simulink model "SeatMdSwtchArbt"  (R2018b)
settings: Solver=FixedStepDiscrete  StartTime=0.0  StopTime=10.0  FixedStep=0.01  RelTol=1e-3
undefined symbols (not defined in the file or in its folder): PosRclRspStat1
libraries: SeatMdSwtchArbt_Lib x35
(part 2 of 2)

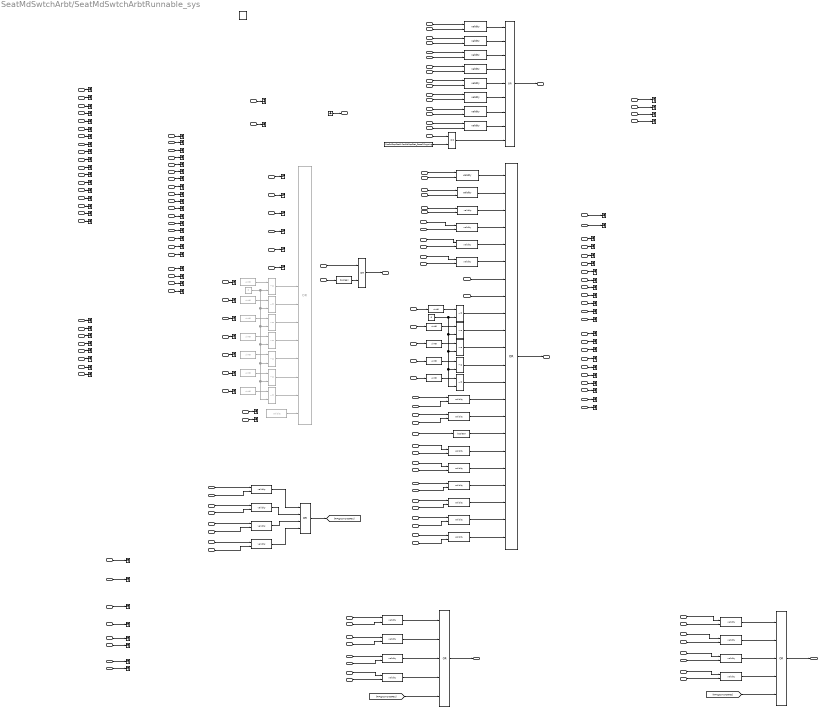
== system SeatMdSwtchArbt/SeatMdSwtchArbtRunnable_sys ==
  note: 2022-02-17:CR202175：修改需求506/548/551/552，新增需求712，完善座椅模式的打断策略。
      | 2023-07-31:增加2L/2R腿托无极调节接口
  note: #尾箱靠背调节
  note: #尾箱前后调节
  note: #坐垫折叠
  IfDrvSeatMemSwtAct1_Val_read : Inport
  IfDrvSeatMemSwtActV1_Val_read : Inport  Port=2
  IfVeSMSb_DrvStCshnRrDnwdMovSwAct_Val_read : Inport  Port=3
  IfVeSMSb_DrvStCshnRrDnwdMovSwActV_Val_read : Inport  Port=4
  IfVeSMSb2LBkReclnSwReq_Val_read : Inport  Port=5
  IfVeSMSb2LBkReclnSwReqV_Val_read : Inport  Port=6
  IfVeSMSb2LSecRwStBkReclnDnwdSwActv_Val_read : Inport  Port=7
  IfVeSMSb2LSecRwStBkReclnUpwdSwActv_Val_read : Inport  Port=8
  IfVeSMSb2LSecRwStBkwdSwActv_Val_read : Inport  Port=9
  IfVeSMSb2LSecRwStFrwdSwActv_Val_read : Inport  Port=10
  IfVeSMSb2LSecRwStLgrstDnwdSwActv_Val_read : Inport  Port=11
  IfVeSMSb2LSecRwStLgrstUpwdSwActv_Val_read : Inport  Port=12
  IfVeSMSbBosSWBkwdHMI2RReq_Val_read : Inport  Port=13
  IfVeSMSbBosSWFrwdHMI2RReq_Val_read : Inport  Port=14
  IfVeSMSbBosSWStBkReclnDnwdHMI2RReq_Val_read : Inport  Port=15
  IfVeSMSbBosSWStBkReclnUpwdHMI2RReq_Val_read : Inport  Port=16
  IfVeSMSbDrvStBkReclnDnwdMovSwAct_Val_read : Inport  Port=17
  IfVeSMSbDrvStBkReclnDnwdMovSwActV_Val_read : Inport  Port=18
  IfVeSMSbDrvStBkReclnUpwdMovSwAct_Val_read : Inport  Port=19
  IfVeSMSbDrvStBkReclnUpwdMovSwActV_Val_read : Inport  Port=20
  IfVeSMSbDrvStBkwdMovSwAct_Val_read : Inport  Port=21
  IfVeSMSbDrvStBkwdMovSwActV_Val_read : Inport  Port=22
  IfVeSMSbDrvStCshnFrntDnwdMovSwAct_Val_read : Inport  Port=23
  IfVeSMSbDrvStCshnFrntDnwdMovSwActV_Val_read : Inport  Port=24
  IfVeSMSbDrvStCshnFrntUpwdMovSwAct_Val_read : Inport  Port=25
  IfVeSMSbDrvStCshnFrntUpwdMovSwActV_Val_read : Inport  Port=26
  IfVeSMSbDrvStCshnRrUpwdMovSwAct_Val_read : Inport  Port=27
  IfVeSMSbDrvStCshnRrUpwdMovSwActV_Val_read : Inport  Port=28
  IfVeSMSbDrvStFrwdMovSwAct_Val_read : Inport  Port=29
  IfVeSMSbDrvStFrwdMovSwActV_Val_read : Inport  Port=30
  IfVeSMSbPassStBkReclnDnwdMovSwAct_Val_read : Inport  Port=31
  IfVeSMSbPassStBkReclnDnwdMovSwActV_Val_read : Inport  Port=32
  IfVeSMSbPassStBkReclnUpwdMovSwAct_Val_read : Inport  Port=33
  IfVeSMSbPassStBkReclnUpwdMovSwActV_Val_read : Inport  Port=34
  IfVeSMSbPassStBkwdMovSwAct_Val_read : Inport  Port=35
  IfVeSMSbPassStBkwdMovSwActV_Val_read : Inport  Port=36
  IfVeSMSbPassStCshnFrntDnwdMovSwAct_Val_read : Inport  Port=37
  IfVeSMSbPassStCshnFrntDnwdMovSwActV_Val_read : Inport  Port=38
  IfVeSMSbPassStCshnFrntUpwdMovSwAct_Val_read : Inport  Port=39
  IfVeSMSbPassStCshnFrntUpwdMovSwActV_Val_read : Inport  Port=40
  IfVeSMSbPassStCshnRrDnwdMovSwAct_Val_read : Inport  Port=41
  IfVeSMSbPassStCshnRrDnwdMovSwActV_Val_read : Inport  Port=42
  IfVeSMSbPassStCshnRrUpwdMovSwAct_Val_read : Inport  Port=43
  IfVeSMSbPassStCshnRrUpwdMovSwActV_Val_read : Inport  Port=44
  IfVeSMSbPassStFrwdMovSwAct_Val_read : Inport  Port=45
  IfVeSMSbPassStFrwdMovSwActV_Val_read : Inport  Port=46
  IfVeSMSbRrLtStFtDnwdHMI2LReq_Val_read : Inport  Port=47
  IfVeSMSbRrLtStFtUpwdHMI2LReq_Val_read : Inport  Port=48
  IfVeSMSbRrPsgComprtStBkReclnDnwdSwReq_Val_read : Inport  Port=49
  IfVeSMSbRrPsgComprtStBkReclnDnwdSwReqV_Val_read : Inport  Port=50
  IfVeSMSbRrPsgComprtStBkReclnUpwdSwReq_Val_read : Inport  Port=51
  IfVeSMSbRrPsgComprtStBkReclnUpwdSwReqV_Val_read : Inport  Port=52
  IfVeSMSbRrPsgComprtStBkwdSwReq_Val_read : Inport  Port=53
  IfVeSMSbRrPsgComprtStBkwdSwReqV_Val_read : Inport  Port=54
  IfVeSMSbRrPsgComprtStFrwdSwReq_Val_read : Inport  Port=55
  IfVeSMSbRrPsgComprtStFrwdSwReqV_Val_read : Inport  Port=56
  IfVeSMSbRrRtStFtDnwdHMI2RReq_Val_read : Inport  Port=57
  IfVeSMSbRrRtStFtUpwdHMI2RReq_Val_read : Inport  Port=58
  IfVeSMSbSecRwLtStArmScrnHMI2LReq_Val_read : Inport  Port=59
  IfVeSMSbSecRwLtStBkReclnDnwdHMI2LReq_Val_read : Inport  Port=60
  IfVeSMSbSecRwLtStBkReclnUpwdHMI2LReq_Val_read : Inport  Port=61
  IfVeSMSbSecRwLtStBkwdHMI2LReq_Val_read : Inport  Port=62
  IfVeSMSbSecRwLtStFrwdHMI2LReq_Val_read : Inport  Port=63
  IfVeSMSbSecRwLtStFtDnwdHMI2LReq_Val_read : Inport  Port=64
  IfVeSMSbSecRwLtStFtUpwdHMI2LReq_Val_read : Inport  Port=65
  IfVeSMSbSecRwLtStHdrstBkwdHMI2LReq_Val_read : Inport  Port=66
  IfVeSMSbSecRwLtStHdrstDnwdHMI2LReq_Val_read : Inport  Port=67
  IfVeSMSbSecRwLtStHdrstFrwdHMI2LReq_Val_read : Inport  Port=68
  IfVeSMSbSecRwLtStHdrstUpwdHMI2LReq_Val_read : Inport  Port=69
  IfVeSMSbSecRwLtStLcMovActv_Val_read : Inport  Port=70
  IfVeSMSbSecRwLtStLgrstDnwdHMI2LReq_Val_read : Inport  Port=71
  IfVeSMSbSecRwLtStLgrstInwdHMI2LReq_Val_read : Inport  Port=72
  IfVeSMSbSecRwLtStLgrstOtwdHMI2LReq_Val_read : Inport  Port=73
  IfVeSMSbSecRwLtStLgrstUpwdHMI2LReq_Val_read : Inport  Port=74
  IfVeSMSbSecRwLtStLtwdHMI2LReq_Val_read : Inport  Port=75
  IfVeSMSbSecRwLtStRtwdHMI2LReq_Val_read : Inport  Port=76
  IfVeSMSbSecRwRtStArmScrnHMI2RReq_Val_read : Inport  Port=77
  IfVeSMSbSecRwRtStBkReclnDnwdHMI2RReq_Val_read : Inport  Port=78
  IfVeSMSbSecRwRtStBkReclnDnwdSwReq_Val_read : Inport  Port=79
  IfVeSMSbSecRwRtStBkReclnDnwdSwReqV_Val_read : Inport  Port=80
  IfVeSMSbSecRwRtStBkReclnUpwdHMI2RReq_Val_read : Inport  Port=81
  IfVeSMSbSecRwRtStBkReclnUpwdSwReq_Val_read : Inport  Port=82
  IfVeSMSbSecRwRtStBkReclnUpwdSwReqV_Val_read : Inport  Port=83
  IfVeSMSbSecRwRtStBkwdHMI2RReq_Val_read : Inport  Port=84
  IfVeSMSbSecRwRtStBkwdSwReq_Val_read : Inport  Port=85
  IfVeSMSbSecRwRtStBkwdSwReqV_Val_read : Inport  Port=86
  IfVeSMSbSecRwRtStFrwdHMI2RReq_Val_read : Inport  Port=87
  IfVeSMSbSecRwRtStFrwdSwReq_Val_read : Inport  Port=88
  IfVeSMSbSecRwRtStFrwdSwReqV_Val_read : Inport  Port=89
  IfVeSMSbSecRwRtStFtDnwdHMI2RReq_Val_read : Inport  Port=90
  IfVeSMSbSecRwRtStFtUpwdHMI2RReq_Val_read : Inport  Port=91
  IfVeSMSbSecRwRtStHdrstBkwdHMI2RReq_Val_read : Inport  Port=92
  IfVeSMSbSecRwRtStHdrstDnwdHMI2RReq_Val_read : Inport  Port=93
  IfVeSMSbSecRwRtStHdrstFrwdHMI2RReq_Val_read : Inport  Port=94
  IfVeSMSbSecRwRtStHdrstUpwdHMI2RReq_Val_read : Inport  Port=95
  IfVeSMSbSecRwRtStLgrstDnwdHMI2RReq_Val_read : Inport  Port=96
  IfVeSMSbSecRwRtStLgrstDnwdSwReq_Val_read : Inport  Port=97
  IfVeSMSbSecRwRtStLgrstDnwdSwReqV_Val_read : Inport  Port=98
  IfVeSMSbSecRwRtStLgrstInwdHMI2RReq_Val_read : Inport  Port=99
  IfVeSMSbSecRwRtStLgrstOtwdHMI2RReq_Val_read : Inport  Port=100
  IfVeSMSbSecRwRtStLgrstUpwdHMI2RReq_Val_read : Inport  Port=101
  IfVeSMSbSecRwRtStLgrstUpwdSwReq_Val_read : Inport  Port=102
  IfVeSMSbSecRwRtStLgrstUpwdSwReqV_Val_read : Inport  Port=103
  IfVeSMSbSecRwRtStLmbrHMI2RReq_Val_read : Inport  Port=104
  IfVeSMSbSecRwRtStLtwdHMI2RReq_Val_read : Inport  Port=105
  IfVeSMSbSecRwRtStRtwdHMI2RReq_Val_read : Inport  Port=106
  IfVeSMSbThdRLtStExpdSwReq_Val_read : Inport  Port=107
  IfVeSMSbThdRLtStExpdSwReqV_Val_read : Inport  Port=108
  IfVeSMSbThdRRtStExpdSwReq_Val_read : Inport  Port=109
  IfVeSMSbThdRRtStExpdSwReqV_Val_read : Inport  Port=110
  IfVeSMSbThdRwLtStBkReclnDnwdSwReq_Val_read : Inport  Port=111
  IfVeSMSbThdRwLtStBkReclnDnwdSwReqV_Val_read : Inport  Port=112
  IfVeSMSbThdRwLtStBkReclnUpwdSwReq_Val_read : Inport  Port=113
  IfVeSMSbThdRwLtStBkReclnUpwdSwReqV_Val_read : Inport  Port=114
  IfVeSMSbThdRwLtStBkwdSwReq_Val_read : Inport  Port=115
  IfVeSMSbThdRwLtStBkwdSwReqV_Val_read : Inport  Port=116
  IfVeSMSbThdRwLtStFrwdSwReq_Val_read : Inport  Port=117
  IfVeSMSbThdRwLtStFrwdSwReqV_Val_read : Inport  Port=118
  IfVeSMSbThdRwRtStBkReclnDnwdSwReq_Val_read : Inport  Port=119
  IfVeSMSbThdRwRtStBkReclnDnwdSwReqV_Val_read : Inport  Port=120
  IfVeSMSbThdRwRtStBkReclnUpwdSwReq_Val_read : Inport  Port=121
  IfVeSMSbThdRwRtStBkReclnUpwdSwReqV_Val_read : Inport  Port=122
  IfVeSMSbThdRwRtStBkwdSwReq_Val_read : Inport  Port=123
  IfVeSMSbThdRwRtStBkwdSwReqV_Val_read : Inport  Port=124
  IfVeSMSbThdRwRtStFrwdSwReq_Val_read : Inport  Port=125
  IfVeSMSbThdRwRtStFrwdSwReqV_Val_read : Inport  Port=126
  IfVeSMSeSecLTMemHMI2LReq1_Val_read : Inport  Port=127
  IfVeSMSeSecLTMemHMI2RReq1_Val_read : Inport  Port=128
  IfVeSMSuSeatPosEnable_Val_read : Inport  Port=129
  StSlctSwReq_Val_read : Inport  Port=130
  StSlctSwReqV_Val_read : Inport  Port=131
  IfVeSMSuRrLtStFtUpwdPstnHMI2LReq_Val_read : Inport  Port=132
  IfVeSMSuRrLtStFtUpwdPstnHMI2LReqV_Val_read : Inport  Port=133
  IfVeSMSuRrRtStFtUpwdPstnHMI2RReq_Val_read : Inport  Port=134
  IfVeSMSuRrRtStFtUpwdPstnHMI2RReqV_Val_read : Inport  Port=135
  IfVeSMSbSecRwLtStFtClsHMI2LReq_Val_read : Inport  Port=136
  IfVeSMSbSecRwLtStFtOpenHMI2LReq_Val_read : Inport  Port=137
  IfVeSMSbSecRwRtStFtClsHMI2LReq_Val_read : Inport  Port=138
  IfVeSMSbSecRwRtStFtOpenHMI2LReq_Val_read : Inport  Port=139
  IfSecRwLtStCushnFrtDnwdHMI2LReq_Val_read : Inport  Port=140
  IfSecRwLtStCushnFrtUpwdDnwdMovmtVirtCtrlReq_Val_read : Inport  Port=141
  IfSecRwLtStCushnFrtUpwdHMI2LReq_Val_read : Inport  Port=142
  IfSecRwLtStFwdBkwdMovmtVirtCtrlReq_Val_read : Inport  Port=143
  IfSecRwLtStLgrstOtwdInwdMovmtVirtCtrlReq_Val_read : Inport  Port=144
  IfSecRwLtStLgrstUpwdDnwdMovmtVirtCtrlReq_Val_read : Inport  Port=145
  IfSecRwLtStRclUpwdDnwdMovmtVirtCtrlReq_Val_read : Inport  Port=146
  IfSecRwRtStCushnFrtDnwdHMI2LReq_Val_read : Inport  Port=147
  IfSecRwRtStCushnFrtUpwdDnwdMovmtVirtCtrlReq_Val_read : Inport  Port=148
  IfSecRwRtStCushnFrtUpwdHMI2LReq_Val_read : Inport  Port=149
  IfSecRwRtStFwdBkwdMovmtVirtCtrlReq_Val_read : Inport  Port=150
  IfSecRwRtStLgrstOtwdInwdMovmtVirtCtrlReq_Val_read : Inport  Port=151
  IfSecRwRtStLgrstUpwdDnwdMovmtVirtCtrlReq_Val_read : Inport  Port=152
  IfSecRwRtStRclUpwdDnwdMovmtVirtCtrlReq_Val_read : Inport  Port=153
  IfSecRwRtStLgrstInwdSwReq_Val_read : Inport  Port=154
  IfSecRwRtStLgrstInwdSwReqV_Val_read : Inport  Port=155
  IfSecRwRtStLgrstOtwdSwReq_Val_read : Inport  Port=156
  IfSecRwRtStLgrstOtwdSwReqV_Val_read : Inport  Port=157
  IfVeSMSbPassStBkReclnDnwdMovBosSwAct_Val_read : Inport  Port=158
  IfVeSMSbPassStBkReclnDnwdMovBosSwActV_Val_read : Inport  Port=159
  IfVeSMSbPassStBkReclnUpwdMovBosSwAct_Val_read : Inport  Port=160
  IfVeSMSbPassStBkReclnUpwdMovBosSwActV_Val_read : Inport  Port=161
  IfVeSMSbPassStBkwdMovBosSwAct_Val_read : Inport  Port=162
  IfVeSMSbPassStBkwdMovBosSwActV_Val_read : Inport  Port=163
  IfVeSMSbPassStFrwdMovBosSwAct_Val_read : Inport  Port=164
  IfVeSMSbPassStFrwdMovBosSwActV_Val_read : Inport  Port=165
  IfSecRwRtStZeroGrvyDnwdSwReq_Val_read : Inport  Port=166
  IfSecRwRtStZeroGrvyDnwdSwReqV_Val_read : Inport  Port=167
  IfSecRwRtStZeroGrvyUpwdSwReq_Val_read : Inport  Port=168
  IfSecRwRtStZeroGrvyUpwdSwReqV_Val_read : Inport  Port=169
  SecRwRtStBkReclnDnwdMovBossSwReq_Val_read : Inport  Port=170
  SecRwRtStBkReclnDnwdMovBossSwReqV_Val_read : Inport  Port=171
  SecRwRtStBkReclnUpwdMovBossSwReq_Val_read : Inport  Port=172
  SecRwRtStBkReclnUpwdMovBossSwReqV_Val_read : Inport  Port=173
  SecRwRtStBkwdMovBossSwReq_Val_read : Inport  Port=174
  SecRwRtStBkwdMovBossSwReqV_Val_read : Inport  Port=175
  SecRwRtStFrwdMovBossSwReq_Val_read : Inport  Port=176
  SecRwRtStFrwdMovBossSwReqV_Val_read : Inport  Port=177
  PassStPosRclRspStat_Val_read : Inport  Port=178
  function : TriggerPort  TriggerType=function-call  VariantControl=(inherit)  SampleTimeType=periodic  SampleTime=-1
  AND : Logic  Operator=OR  Inputs=9  AllPortsSameDT=off  OutDataTypeStr=boolean
  Constant1 : Constant  Value=PosRclRspStat1.PosRclRspStat_RecallOngoing  OutDataTypeStr=Enum:PosRclRspStat1
  Constant2 : Constant  Commented=on  Value=0  OutDataTypeStr=uint8
  Constant3 : Constant  Value=0  OutDataTypeStr=uint8
  Data Type Conversion{,1..6} (7 alike) : DataTypeConversion  Commented=on  OutDataTypeStr=uint8
  Data Type Conversion{7..9,11,13} (5 alike) : DataTypeConversion  OutDataTypeStr=uint8
  Data Type Conversion14 : DataTypeConversion  OutDataTypeStr=boolean
  Data Type Conversion15 : DataTypeConversion  OutDataTypeStr=boolean
  Equal{,1..6} (7 alike) : RelationalOperator  Commented=on  Operator=~=  OutDataTypeStr=boolean  RndMeth=Simplest
  Equal10 : RelationalOperator  Operator===  OutDataTypeStr=boolean  RndMeth=Simplest
  Equal{7..9,11,13} (5 alike) : RelationalOperator  Operator=~=  OutDataTypeStr=boolean  RndMeth=Simplest
  Ground : Ground
  Logical Operator1 : Logic  Operator=OR  Inputs=5  AllPortsSameDT=off  OutDataTypeStr=boolean
  Logical Operator19 : Logic  Commented=on  Operator=OR  Inputs=14  AllPortsSameDT=off  OutDataTypeStr=boolean
  Logical Operator26 : Logic  Operator=OR  Inputs=22  AllPortsSameDT=off  OutDataTypeStr=boolean
  Logical Operator27 : Logic  Operator=OR  Inputs=5  AllPortsSameDT=off  OutDataTypeStr=boolean
  OR : Logic  Operator=OR  AllPortsSameDT=off  OutDataTypeStr=boolean
  OR1 : Logic  Operator=OR  Inputs=4  AllPortsSameDT=off  OutDataTypeStr=boolean
  Terminator_{1..34,37..44,47..69,71..72,74..82,84..105,129} (99 alike) : Terminator
  validity{1..6,8..35} (34 alike) : SeatMdSwtchArbt_Lib/validity  SystemSampleTime=-1
  validity7 : SeatMdSwtchArbt_Lib/validity  Commented=on  SystemSampleTime=-1
  IfVeSMSbIs2LStSwAct_Val_write : Outport
  IfVeSMSbIs2RStSwAct_Val_write : Outport  Port=2
  IfVeSMSbIs3LStSwAct_Val_write : Outport  Port=3
  IfVeSMSbIs3RStSwAct_Val_write : Outport  Port=4
  IfVeSMSbIsDrvStSwAct_Val_write : Outport  Port=5
  IfVeSMSbIsPasStSwAct_Val_write : Outport  Port=6
  wires:
  IfDrvSeatMemSwtAct1_Val_read/1 -> Terminator_1/1
  IfDrvSeatMemSwtActV1_Val_read/1 -> Terminator_2/1
  IfVeSMSb_DrvStCshnRrDnwdMovSwAct_Val_read/1 -> Terminator_3/1
  IfVeSMSb_DrvStCshnRrDnwdMovSwActV_Val_read/1 -> Terminator_4/1
  IfVeSMSbDrvStBkReclnDnwdMovSwAct_Val_read/1 -> Terminator_17/1
  IfVeSMSbDrvStBkReclnDnwdMovSwActV_Val_read/1 -> Terminator_18/1
  IfVeSMSbDrvStBkReclnUpwdMovSwAct_Val_read/1 -> Terminator_19/1
  IfVeSMSbDrvStBkReclnUpwdMovSwActV_Val_read/1 -> Terminator_20/1
  IfVeSMSbDrvStBkwdMovSwAct_Val_read/1 -> Terminator_21/1
  IfVeSMSbDrvStBkwdMovSwActV_Val_read/1 -> Terminator_22/1
  IfVeSMSbDrvStCshnFrntDnwdMovSwAct_Val_read/1 -> Terminator_23/1
  IfVeSMSbDrvStCshnFrntDnwdMovSwActV_Val_read/1 -> Terminator_24/1
  IfVeSMSbDrvStCshnFrntUpwdMovSwAct_Val_read/1 -> Terminator_25/1
  IfVeSMSbDrvStCshnFrntUpwdMovSwActV_Val_read/1 -> Terminator_26/1
  IfVeSMSbDrvStCshnRrUpwdMovSwAct_Val_read/1 -> Terminator_27/1
  IfVeSMSbDrvStCshnRrUpwdMovSwActV_Val_read/1 -> Terminator_28/1
  IfVeSMSbDrvStFrwdMovSwAct_Val_read/1 -> Terminator_29/1
  IfVeSMSbDrvStFrwdMovSwActV_Val_read/1 -> Terminator_30/1
  IfVeSMSbPassStCshnFrntDnwdMovSwAct_Val_read/1 -> Terminator_37/1
  IfVeSMSbPassStCshnFrntDnwdMovSwActV_Val_read/1 -> Terminator_38/1
  IfVeSMSbPassStCshnFrntUpwdMovSwAct_Val_read/1 -> Terminator_39/1
  IfVeSMSbPassStCshnFrntUpwdMovSwActV_Val_read/1 -> Terminator_40/1
  IfVeSMSbPassStCshnRrDnwdMovSwAct_Val_read/1 -> Terminator_41/1
  IfVeSMSbPassStCshnRrDnwdMovSwActV_Val_read/1 -> Terminator_42/1
  IfVeSMSbPassStCshnRrUpwdMovSwAct_Val_read/1 -> Terminator_43/1
  IfVeSMSbPassStCshnRrUpwdMovSwActV_Val_read/1 -> Terminator_44/1
  IfVeSMSbSecRwRtStLmbrHMI2RReq_Val_read/1 -> Terminator_104/1
  IfVeSMSuSeatPosEnable_Val_read/1 -> Terminator_129/1
  Ground/1 -> IfVeSMSbIsDrvStSwAct_Val_write/1
  IfVeSMSbSecRwRtStBkReclnUpwdSwReqV_Val_read/1 -> validity19/2
  IfVeSMSbSecRwRtStLgrstDnwdSwReqV_Val_read/1 -> validity22/2
  IfVeSMSbSecRwRtStFrwdSwReq_Val_read/1 -> validity21/1
  IfVeSMSbSecRwRtStLgrstUpwdSwReq_Val_read/1 -> validity23/1
  IfVeSMSbSecRwRtStBkReclnUpwdSwReq_Val_read/1 -> validity19/1
  IfVeSMSbSecRwRtStLgrstUpwdSwReqV_Val_read/1 -> validity23/2
  IfVeSMSbSecRwRtStFrwdSwReqV_Val_read/1 -> validity21/2
  Logical Operator26/1 -> IfVeSMSbIs2RStSwAct_Val_write/1
  IfVeSMSbSecRwRtStBkReclnDnwdSwReq_Val_read/1 -> validity18/1
  IfVeSMSbSecRwRtStBkReclnDnwdSwReqV_Val_read/1 -> validity18/2
  IfVeSMSbSecRwRtStBkwdSwReq_Val_read/1 -> validity20/1
  IfVeSMSbSecRwRtStBkwdSwReqV_Val_read/1 -> validity20/2
  IfVeSMSbSecRwRtStLgrstDnwdSwReq_Val_read/1 -> validity22/1
  IfVeSMSbRrPsgComprtStBkReclnDnwdSwReq_Val_read/1 -> validity3/1
  validity5/1 -> OR1/3
  IfVeSMSbRrPsgComprtStBkReclnDnwdSwReqV_Val_read/1 -> validity3/2
  validity4/1 -> OR1/2
  IfVeSMSbRrPsgComprtStFrwdSwReqV_Val_read/1 -> validity6/2
  IfVeSMSbRrPsgComprtStBkwdSwReqV_Val_read/1 -> validity5/2
  IfVeSMSbRrPsgComprtStFrwdSwReq_Val_read/1 -> validity6/1
  IfVeSMSbRrPsgComprtStBkReclnUpwdSwReq_Val_read/1 -> validity4/1
  IfVeSMSbRrPsgComprtStBkwdSwReq_Val_read/1 -> validity5/1
  validity6/1 -> OR1/4
  OR1/1 -> [RrPsgComprtStReq]
  validity3/1 -> OR1/1
  IfVeSMSbRrPsgComprtStBkReclnUpwdSwReqV_Val_read/1 -> validity4/2
  validity27/1 -> Logical Operator27/4
  IfVeSMSbThdRwLtStBkReclnUpwdSwReq_Val_read/1 -> validity25/1
  IfVeSMSbThdRwLtStBkReclnDnwdSwReqV_Val_read/1 -> validity24/2
  validity24/1 -> Logical Operator27/1
  IfVeSMSbThdRwLtStBkReclnDnwdSwReq_Val_read/1 -> validity24/1
  IfVeSMSbThdRwLtStFrwdSwReqV_Val_read/1 -> validity27/2
  IfVeSMSbThdRwLtStBkReclnUpwdSwReqV_Val_read/1 -> validity25/2
  IfVeSMSbThdRwLtStFrwdSwReq_Val_read/1 -> validity27/1
  validity25/1 -> Logical Operator27/2
  IfVeSMSbThdRwLtStBkwdSwReq_Val_read/1 -> validity26/1
  validity26/1 -> Logical Operator27/3
  Logical Operator27/1 -> IfVeSMSbIs3LStSwAct_Val_write/1
  IfVeSMSbThdRwLtStBkwdSwReqV_Val_read/1 -> validity26/2
  validity17/1 -> Logical Operator1/1
  IfVeSMSbThdRwRtStBkReclnDnwdSwReqV_Val_read/1 -> validity17/2
  validity30/1 -> Logical Operator1/4
  validity29/1 -> Logical Operator1/3
  IfVeSMSbThdRwRtStBkReclnUpwdSwReq_Val_read/1 -> validity28/1
  IfVeSMSbThdRwRtStBkwdSwReq_Val_read/1 -> validity29/1
  IfVeSMSbThdRwRtStBkReclnDnwdSwReq_Val_read/1 -> validity17/1
  IfVeSMSbThdRwRtStBkReclnUpwdSwReqV_Val_read/1 -> validity28/2
  validity28/1 -> Logical Operator1/2
  IfVeSMSbThdRwRtStFrwdSwReq_Val_read/1 -> validity30/1
  Logical Operator1/1 -> IfVeSMSbIs3RStSwAct_Val_write/1
  IfVeSMSbThdRwRtStBkwdSwReqV_Val_read/1 -> validity29/2
  IfVeSMSbThdRwRtStFrwdSwReqV_Val_read/1 -> validity30/2
  StSlctSwReq_Val_read/1 -> Terminator_5/1
  StSlctSwReqV_Val_read/1 -> Terminator_6/1
  IfVeSMSbSecRwLtStFtDnwdHMI2LReq_Val_read/1 -> Terminator_11/1
  IfVeSMSbSecRwLtStFtUpwdHMI2LReq_Val_read/1 -> Terminator_12/1
  IfVeSMSbSecRwRtStFtDnwdHMI2RReq_Val_read/1 -> Terminator_13/1
  IfVeSMSbSecRwRtStFtUpwdHMI2RReq_Val_read/1 -> Terminator_14/1
  IfVeSMSbSecRwLtStBkReclnDnwdHMI2LReq_Val_read/1 -> Terminator_15/1
  IfVeSMSbSecRwLtStBkReclnUpwdHMI2LReq_Val_read/1 -> Terminator_16/1
  IfVeSMSbSecRwLtStFrwdHMI2LReq_Val_read/1 -> Terminator_54/1
  IfVeSMSbSecRwLtStBkwdHMI2LReq_Val_read/1 -> Terminator_47/1
  IfVeSMSbSecRwLtStHdrstUpwdHMI2LReq_Val_read/1 -> Terminator_51/1
  IfVeSMSbSecRwLtStHdrstDnwdHMI2LReq_Val_read/1 -> Terminator_62/1
  IfVeSMSbSecRwLtStLgrstUpwdHMI2LReq_Val_read/1 -> Terminator_63/1
  IfVeSMSbSecRwLtStLgrstDnwdHMI2LReq_Val_read/1 -> Terminator_64/1
  IfVeSMSbSecRwLtStLtwdHMI2LReq_Val_read/1 -> Terminator_53/1
  IfVeSMSbSecRwLtStRtwdHMI2LReq_Val_read/1 -> Terminator_65/1
  IfVeSMSbRrLtStFtDnwdHMI2LReq_Val_read/1 -> Terminator_66/1
  IfVeSMSbRrLtStFtUpwdHMI2LReq_Val_read/1 -> Terminator_67/1
  IfVeSMSbSecRwLtStHdrstBkwdHMI2LReq_Val_read/1 -> Terminator_68/1
  IfVeSMSbSecRwLtStHdrstFrwdHMI2LReq_Val_read/1 -> Terminator_69/1
  IfVeSMSbSecRwLtStLgrstInwdHMI2LReq_Val_read/1 -> Terminator_71/1
  IfVeSMSbSecRwLtStLgrstOtwdHMI2LReq_Val_read/1 -> Terminator_72/1
  IfVeSMSbSecRwLtStArmScrnHMI2LReq_Val_read/1 -> Terminator_52/1
  IfVeSMSuRrLtStFtUpwdPstnHMI2LReq_Val_read/1 -> Terminator_74/1
  IfVeSMSuRrLtStFtUpwdPstnHMI2LReqV_Val_read/1 -> Terminator_75/1
  IfVeSMSbSecRwLtStFtOpenHMI2LReq_Val_read/1 -> Terminator_76/1
  IfVeSMSbSecRwLtStFtClsHMI2LReq_Val_read/1 -> Terminator_77/1
  Equal/1 -> Logical Operator19/7
  Constant2/1 -> Equal2/2, Equal6/2, Equal5/2, Equal4/2, Equal3/2, Equal1/2, Equal/2
  Equal1/1 -> Logical Operator19/8
  Equal2/1 -> Logical Operator19/9
  Equal3/1 -> Logical Operator19/10
  validity7/1 -> Logical Operator19/14
  Equal6/1 -> Logical Operator19/13
  Equal5/1 -> Logical Operator19/12
  Equal4/1 -> Logical Operator19/11
  IfVeSMSbSecRwRtStArmScrnHMI2RReq_Val_read/1 -> Terminator_48/1
  IfVeSMSbSecRwRtStBkReclnUpwdHMI2RReq_Val_read/1 -> Terminator_49/1
  IfVeSMSbSecRwRtStBkReclnDnwdHMI2RReq_Val_read/1 -> Terminator_50/1
  IfVeSMSbSecRwRtStBkwdHMI2RReq_Val_read/1 -> Terminator_61/1
  IfVeSMSbSecRwRtStFrwdHMI2RReq_Val_read/1 -> Terminator_78/1
  validity18/1 -> Logical Operator26/1
  validity19/1 -> Logical Operator26/2
  validity20/1 -> Logical Operator26/3
  validity21/1 -> Logical Operator26/4
  validity22/1 -> Logical Operator26/5
  validity23/1 -> Logical Operator26/6
  Constant3/1 -> Equal13/2, Equal11/2, Equal9/2, Equal8/2, Equal7/2
  IfVeSMSbSecRwRtStHdrstDnwdHMI2RReq_Val_read/1 -> Terminator_58/1
  IfVeSMSbSecRwRtStHdrstUpwdHMI2RReq_Val_read/1 -> Terminator_79/1
  IfVeSMSbSecRwRtStLgrstDnwdHMI2RReq_Val_read/1 -> Terminator_80/1
  IfVeSMSbSecRwRtStLgrstUpwdHMI2RReq_Val_read/1 -> Terminator_81/1
  IfVeSMSbSecRwRtStLtwdHMI2RReq_Val_read/1 -> Terminator_60/1
  IfVeSMSbSecRwRtStRtwdHMI2RReq_Val_read/1 -> Terminator_82/1
  IfVeSMSbRrRtStFtDnwdHMI2RReq_Val_read/1 -> Terminator_84/1
  IfVeSMSbRrRtStFtUpwdHMI2RReq_Val_read/1 -> Terminator_85/1
  IfVeSMSbSecRwRtStHdrstBkwdHMI2RReq_Val_read/1 -> Terminator_86/1
  IfVeSMSbSecRwRtStHdrstFrwdHMI2RReq_Val_read/1 -> Terminator_87/1
  IfVeSMSbSecRwRtStLgrstInwdHMI2RReq_Val_read/1 -> Terminator_88/1
  IfVeSMSbSecRwRtStLgrstOtwdHMI2RReq_Val_read/1 -> Terminator_89/1
  IfVeSMSuRrRtStFtUpwdPstnHMI2RReq_Val_read/1 -> Terminator_90/1
  IfVeSMSuRrRtStFtUpwdPstnHMI2RReqV_Val_read/1 -> Terminator_91/1
  IfVeSMSbSecRwRtStFtOpenHMI2LReq_Val_read/1 -> Terminator_92/1
  IfVeSMSbSecRwRtStFtClsHMI2LReq_Val_read/1 -> Terminator_93/1
  Data Type Conversion/1 -> Equal/1
  Data Type Conversion1/1 -> Equal1/1
  Data Type Conversion2/1 -> Equal2/1
  Data Type Conversion3/1 -> Equal3/1
  Data Type Conversion4/1 -> Equal4/1
  Data Type Conversion5/1 -> Equal5/1
  Data Type Conversion6/1 -> Equal6/1
  Data Type Conversion7/1 -> Equal7/1
  IfSecRwRtStRclUpwdDnwdMovmtVirtCtrlReq_Val_read/1 -> Data Type Conversion7/1
  Data Type Conversion8/1 -> Equal8/1
  IfSecRwRtStFwdBkwdMovmtVirtCtrlReq_Val_read/1 -> Data Type Conversion8/1
  Data Type Conversion9/1 -> Equal9/1
  IfSecRwRtStLgrstUpwdDnwdMovmtVirtCtrlReq_Val_read/1 -> Data Type Conversion9/1
  Data Type Conversion11/1 -> Equal11/1
  IfSecRwRtStCushnFrtUpwdDnwdMovmtVirtCtrlReq_Val_read/1 -> Data Type Conversion11/1
  Data Type Conversion13/1 -> Equal13/1
  IfSecRwRtStLgrstOtwdInwdMovmtVirtCtrlReq_Val_read/1 -> Data Type Conversion13/1
  IfVeSMSb2LSecRwStBkReclnDnwdSwActv_Val_read/1 -> Terminator_55/1
  IfVeSMSb2LSecRwStBkReclnUpwdSwActv_Val_read/1 -> Terminator_56/1
  IfVeSMSb2LSecRwStBkwdSwActv_Val_read/1 -> Terminator_57/1
  IfVeSMSb2LSecRwStFrwdSwActv_Val_read/1 -> Terminator_59/1
  IfVeSMSb2LSecRwStLgrstDnwdSwActv_Val_read/1 -> Terminator_94/1
  IfVeSMSb2LSecRwStLgrstUpwdSwActv_Val_read/1 -> Terminator_95/1
  IfSecRwLtStRclUpwdDnwdMovmtVirtCtrlReq_Val_read/1 -> Terminator_96/1
  IfSecRwLtStFwdBkwdMovmtVirtCtrlReq_Val_read/1 -> Terminator_97/1
  IfSecRwLtStLgrstUpwdDnwdMovmtVirtCtrlReq_Val_read/1 -> Terminator_98/1
  IfSecRwLtStLgrstOtwdInwdMovmtVirtCtrlReq_Val_read/1 -> Terminator_99/1
  IfSecRwLtStCushnFrtDnwdHMI2LReq_Val_read/1 -> Terminator_100/1
  IfSecRwLtStCushnFrtUpwdDnwdMovmtVirtCtrlReq_Val_read/1 -> Terminator_101/1
  IfSecRwLtStCushnFrtUpwdHMI2LReq_Val_read/1 -> Terminator_102/1
  IfVeSMSb2LBkReclnSwReq_Val_read/1 -> Terminator_103/1
  IfVeSMSb2LBkReclnSwReqV_Val_read/1 -> Terminator_105/1
  IfVeSMSeSecLTMemHMI2LReq1_Val_read/1 -> Data Type Conversion14/1
  IfVeSMSbSecRwLtStLcMovActv_Val_read/1 -> OR/1
  Data Type Conversion14/1 -> OR/2
  OR/1 -> IfVeSMSbIs2LStSwAct_Val_write/1
  IfVeSMSeSecLTMemHMI2RReq1_Val_read/1 -> Data Type Conversion15/1
  Equal13/1 -> Logical Operator26/13
  Equal11/1 -> Logical Operator26/12
  Equal9/1 -> Logical Operator26/11
  Equal8/1 -> Logical Operator26/10
  Equal7/1 -> Logical Operator26/9
  IfSecRwRtStCushnFrtDnwdHMI2LReq_Val_read/1 -> Logical Operator26/7
  IfSecRwRtStCushnFrtUpwdHMI2LReq_Val_read/1 -> Logical Operator26/8
  IfSecRwRtStLgrstInwdSwReq_Val_read/1 -> validity8/1
  IfSecRwRtStLgrstInwdSwReqV_Val_read/1 -> validity8/2
  validity8/1 -> Logical Operator26/14
  validity9/1 -> Logical Operator26/15
  IfSecRwRtStLgrstOtwdSwReq_Val_read/1 -> validity9/1
  IfSecRwRtStLgrstOtwdSwReqV_Val_read/1 -> validity9/2
  Data Type Conversion15/1 -> Logical Operator26/16
  IfVeSMSbPassStFrwdMovSwAct_Val_read/1 -> validity10/1
  IfVeSMSbPassStFrwdMovSwActV_Val_read/1 -> validity10/2
  IfVeSMSbPassStBkwdMovSwAct_Val_read/1 -> validity11/1
  IfVeSMSbPassStBkwdMovSwActV_Val_read/1 -> validity11/2
  IfVeSMSbPassStBkReclnDnwdMovSwActV_Val_read/1 -> validity12/2
  IfVeSMSbPassStBkReclnDnwdMovSwAct_Val_read/1 -> validity12/1
  IfVeSMSbPassStBkReclnUpwdMovSwAct_Val_read/1 -> validity13/1
  IfVeSMSbPassStBkReclnUpwdMovSwActV_Val_read/1 -> validity13/2
  validity10/1 -> AND/1
  validity11/1 -> AND/2
  validity12/1 -> AND/3
  validity13/1 -> AND/4
  AND/1 -> IfVeSMSbIsPasStSwAct_Val_write/1
  IfVeSMSbThdRLtStExpdSwReq_Val_read/1 -> Terminator_7/1
  IfVeSMSbThdRLtStExpdSwReqV_Val_read/1 -> Terminator_8/1
  IfVeSMSbBosSWFrwdHMI2RReq_Val_read/1 -> Terminator_9/1
  IfVeSMSbBosSWBkwdHMI2RReq_Val_read/1 -> Terminator_10/1
  IfVeSMSbBosSWStBkReclnDnwdHMI2RReq_Val_read/1 -> Terminator_31/1
  IfVeSMSbBosSWStBkReclnUpwdHMI2RReq_Val_read/1 -> Terminator_32/1
  IfVeSMSbThdRRtStExpdSwReq_Val_read/1 -> Terminator_33/1
  IfVeSMSbThdRRtStExpdSwReqV_Val_read/1 -> Terminator_34/1
  [RrPsgComprtStReq] -> Logical Operator27/5
  [RrPsgComprtStReq] -> Logical Operator1/5
  IfVeSMSbPassStBkReclnDnwdMovBosSwAct_Val_read/1 -> validity1/1
  IfVeSMSbPassStBkReclnDnwdMovBosSwActV_Val_read/1 -> validity1/2
  IfVeSMSbPassStBkReclnUpwdMovBosSwAct_Val_read/1 -> validity2/1
  IfVeSMSbPassStBkReclnUpwdMovBosSwActV_Val_read/1 -> validity2/2
  IfVeSMSbPassStBkwdMovBosSwAct_Val_read/1 -> validity14/1
  IfVeSMSbPassStBkwdMovBosSwActV_Val_read/1 -> validity14/2
  IfVeSMSbPassStFrwdMovBosSwAct_Val_read/1 -> validity15/1
  IfVeSMSbPassStFrwdMovBosSwActV_Val_read/1 -> validity15/2
  validity1/1 -> AND/5
  validity2/1 -> AND/6
  validity14/1 -> AND/7
  validity15/1 -> AND/8
  validity16/1 -> Logical Operator26/17
  IfSecRwRtStZeroGrvyDnwdSwReq_Val_read/1 -> validity16/1
  IfSecRwRtStZeroGrvyDnwdSwReqV_Val_read/1 -> validity16/2
  validity31/1 -> Logical Operator26/18
  IfSecRwRtStZeroGrvyUpwdSwReqV_Val_read/1 -> validity31/2
  IfSecRwRtStZeroGrvyUpwdSwReq_Val_read/1 -> validity31/1
  SecRwRtStBkReclnDnwdMovBossSwReq_Val_read/1 -> validity32/1
  SecRwRtStBkReclnDnwdMovBossSwReqV_Val_read/1 -> validity32/2
  SecRwRtStBkReclnUpwdMovBossSwReq_Val_read/1 -> validity33/1
  SecRwRtStBkReclnUpwdMovBossSwReqV_Val_read/1 -> validity33/2
  SecRwRtStBkwdMovBossSwReq_Val_read/1 -> validity34/1
  SecRwRtStBkwdMovBossSwReqV_Val_read/1 -> validity34/2
  SecRwRtStFrwdMovBossSwReq_Val_read/1 -> validity35/1
  SecRwRtStFrwdMovBossSwReqV_Val_read/1 -> validity35/2
  validity32/1 -> Logical Operator26/19
  validity35/1 -> Logical Operator26/22
  validity34/1 -> Logical Operator26/21
  validity33/1 -> Logical Operator26/20
  PassStPosRclRspStat_Val_read/1 -> Equal10/1
  Constant1/1 -> Equal10/2
  Equal10/1 -> AND/9

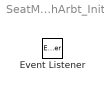
== system SeatMdSwtchArbt/SeatMdSwtchArbt_Init ==
  Event Listener : EventListener  EventName=reset
